simulink model "paper_model"  (R2021a)
settings: Solver=VariableStepAuto  StartTime=0.0  StopTime=720  RelTol=1e-3
libraries: fuzblock x2, mpcadaslib x1
settings Model: Creator=uddin  LastModifiedBy=uddin

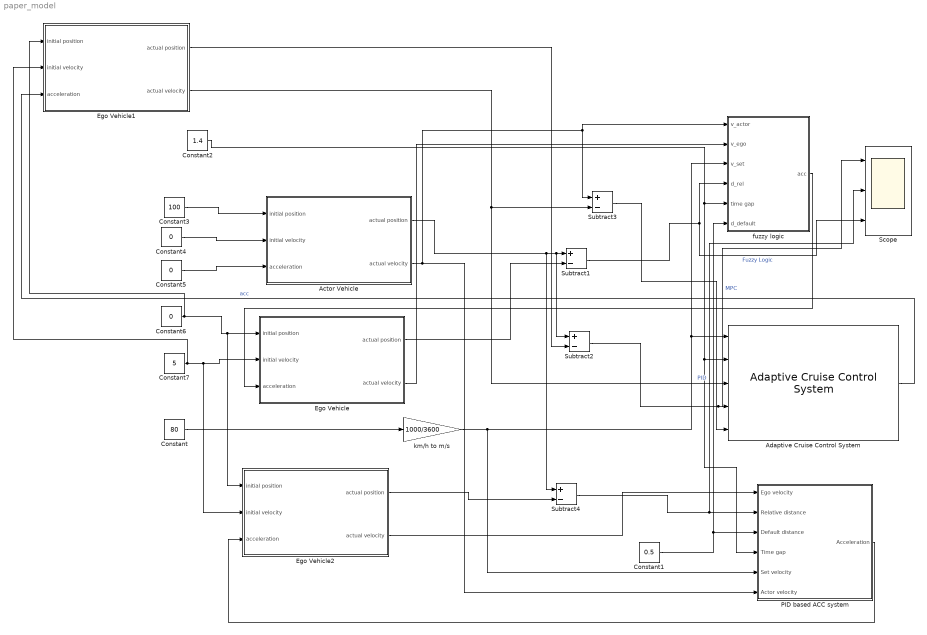
== system paper_model ==
  Actor Vehicle : Subsystem
  Adaptive Cruise Control System : mpcadaslib/Adaptive Cruise Control System  EgoModel=tf(1,[0.5,1,0])  InitialEgoVelocity=50*1000/3600  DefaultSpacing=0.5  MaxVelocity=120*1000/3600  MinAcceleration=-3  amin_ext=off  MaxAcceleration=2  amax_ext=off  Ts=.1  PredictionHorizon=100  ControllerBehavior=0.0  suboptimal=off  maxiter=10  datatypeopt=double  optmode=off  trackmode=off
  Constant : Constant  Value=80
  Constant1 : Constant  Value=0.5  SampleTime=-1
  Constant2 : Constant  Value=1.4  SampleTime=-1
  Constant3 : Constant  Value=100  SampleTime=-1
  Constant4 : Constant  Value=0  SampleTime=-1
  Constant5 : Constant  Value=0  SampleTime=-1
  Constant6 : Constant  Value=0  SampleTime=-1
  Constant7 : Constant  Value=5  SampleTime=-1
  Ego Vehicle : Subsystem
  Ego Vehicle1 : Subsystem
  Ego Vehicle2 : Subsystem
  PID based ACC system : Subsystem
  Scope : Scope  NumInputPorts=3
  Subtract{1..4} (4 alike) : Sum  Inputs=+-
  fuzzy logic : Subsystem
  km/h to m/s : Gain  Gain=1000/3600
  wires:
  Constant5/1 -> Actor Vehicle/3(acceleration)
  Constant3/1 -> Actor Vehicle/1(initial position)
  Constant6/1 -> Ego Vehicle1/1(initial position), Ego Vehicle2/1(initial position), Ego Vehicle/1(initial position)
  Constant7/1 -> Ego Vehicle1/2(initial velocity), Ego Vehicle2/2(initial velocity), Ego Vehicle/2(initial velocity)
  Constant4/1 -> Actor Vehicle/2(initial velocity)
  Actor Vehicle/1(actual position) -> Subtract4/1, Subtract2/1, Subtract1/1
  Actor Vehicle/2(actual velocity) -> PID based ACC system/6(Actor velocity), Subtract3/1, fuzzy logic/1(v_actor)
  Ego Vehicle/1(actual position) -> Subtract1/2
  fuzzy logic/1(acc) -> Ego Vehicle/3(acceleration)
  Subtract1/1 -> Scope/3, fuzzy logic/4(d_rel)  "Fuzzy Logic"
  Constant2/1 -> Adaptive Cruise Control System/2, PID based ACC system/4(Time gap), fuzzy logic/5(time gap)
  Constant/1 -> km/h to m/s/1
  km/h to m/s/1 -> PID based ACC system/5(Set velocity), Adaptive Cruise Control System/1, fuzzy logic/3(v_set)
  Ego Vehicle/2(actual velocity) -> fuzzy logic/2(v_ego)
  Ego Vehicle1/1(actual position) -> Subtract2/2
  Subtract2/1 -> Scope/1, Adaptive Cruise Control System/4  "MPC"
  Ego Vehicle1/2(actual velocity) -> Subtract3/2, Adaptive Cruise Control System/3
  Subtract3/1 -> Adaptive Cruise Control System/5
  Adaptive Cruise Control System/1 -> Ego Vehicle1/3(acceleration)  "acc"
  Ego Vehicle2/1(actual position) -> Subtract4/2
  Subtract4/1 -> PID based ACC system/2(Relative distance), Scope/2  "PID"
  PID based ACC system/1(Acceleration) -> Ego Vehicle2/3(acceleration)
  Ego Vehicle2/2(actual velocity) -> PID based ACC system/1(Ego velocity)
  Constant1/1 -> fuzzy logic/6(d_default), PID based ACC system/3(Default distance)

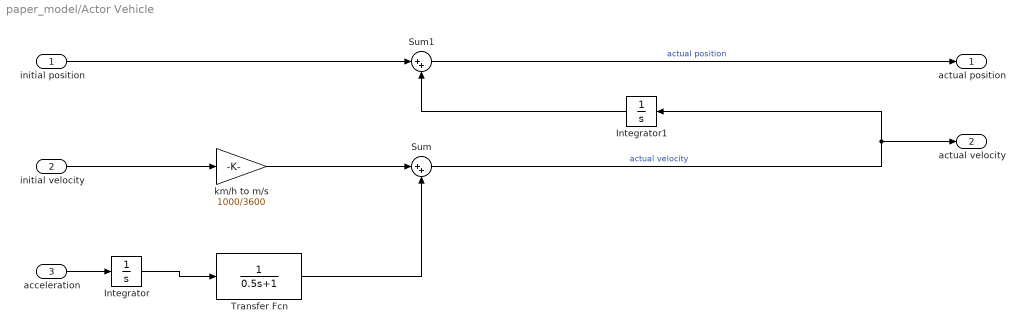
== system paper_model/Actor Vehicle ==
  initial position : Inport
  initial velocity : Inport  Port=2
  acceleration : Inport  Port=3
  Integrator : Integrator
  Integrator1 : Integrator
  Sum : Sum  Inputs=|++
  Sum1 : Sum  Inputs=|++
  Transfer Fcn : TransferFcn  Denominator=[0.5 1]
  km/h to m/s : Gain  Gain=1000/3600
  actual position : Outport
  actual velocity : Outport  Port=2
  wires:
  km/h to m/s/1 -> Sum/1
  initial velocity/1 -> km/h to m/s/1
  Transfer Fcn/1 -> Sum/2
  Integrator/1 -> Transfer Fcn/1
  Integrator1/1 -> Sum1/2
  initial position/1 -> Sum1/1
  acceleration/1 -> Integrator/1
  Sum/1 -> Integrator1/1, actual velocity/1  "actual velocity"
  Sum1/1 -> actual position/1  "actual position"

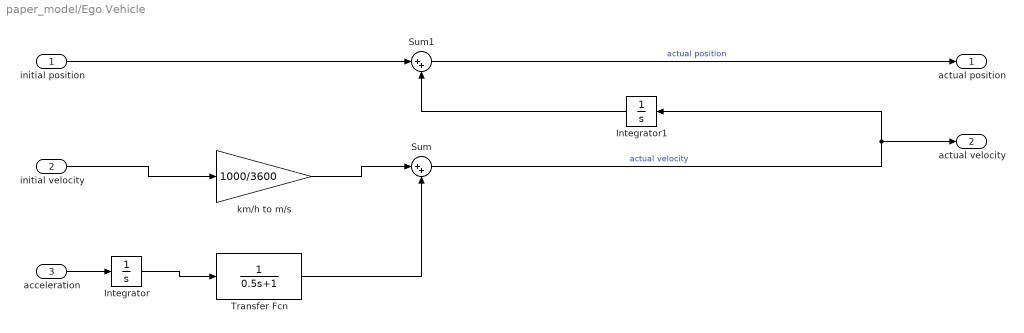
== system paper_model/Ego Vehicle ==
  initial position : Inport
  initial velocity : Inport  Port=2
  acceleration : Inport  Port=3
  Integrator : Integrator
  Integrator1 : Integrator
  Sum : Sum  Inputs=|++
  Sum1 : Sum  Inputs=|++
  Transfer Fcn : TransferFcn  Denominator=[0.5 1]
  km/h to m/s : Gain  Gain=1000/3600
  actual position : Outport
  actual velocity : Outport  Port=2
  wires:
  Sum1/1 -> actual position/1  "actual position"
  Sum/1 -> actual velocity/1, Integrator1/1  "actual velocity"
  acceleration/1 -> Integrator/1
  initial position/1 -> Sum1/1
  Integrator1/1 -> Sum1/2
  Integrator/1 -> Transfer Fcn/1
  Transfer Fcn/1 -> Sum/2
  initial velocity/1 -> km/h to m/s/1
  km/h to m/s/1 -> Sum/1

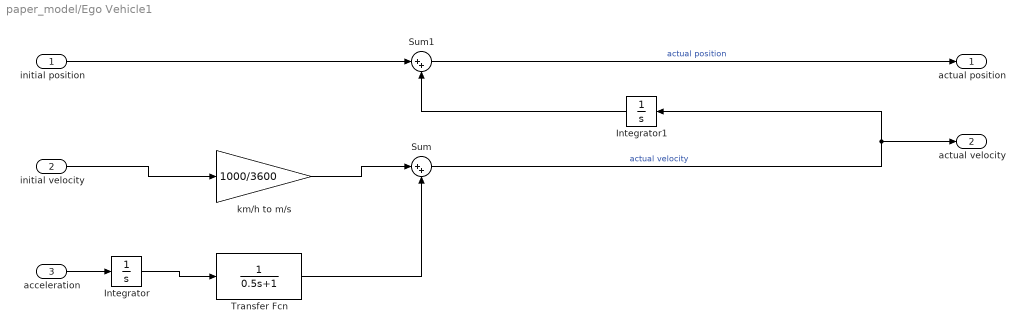
== system paper_model/Ego Vehicle1 ==
  initial position : Inport
  initial velocity : Inport  Port=2
  acceleration : Inport  Port=3
  Integrator : Integrator
  Integrator1 : Integrator
  Sum : Sum  Inputs=|++
  Sum1 : Sum  Inputs=|++
  Transfer Fcn : TransferFcn  Denominator=[0.5 1]
  km/h to m/s : Gain  Gain=1000/3600
  actual position : Outport
  actual velocity : Outport  Port=2
  wires:
  km/h to m/s/1 -> Sum/1
  initial velocity/1 -> km/h to m/s/1
  Transfer Fcn/1 -> Sum/2
  Integrator/1 -> Transfer Fcn/1
  Integrator1/1 -> Sum1/2
  initial position/1 -> Sum1/1
  acceleration/1 -> Integrator/1
  Sum/1 -> Integrator1/1, actual velocity/1  "actual velocity"
  Sum1/1 -> actual position/1  "actual position"

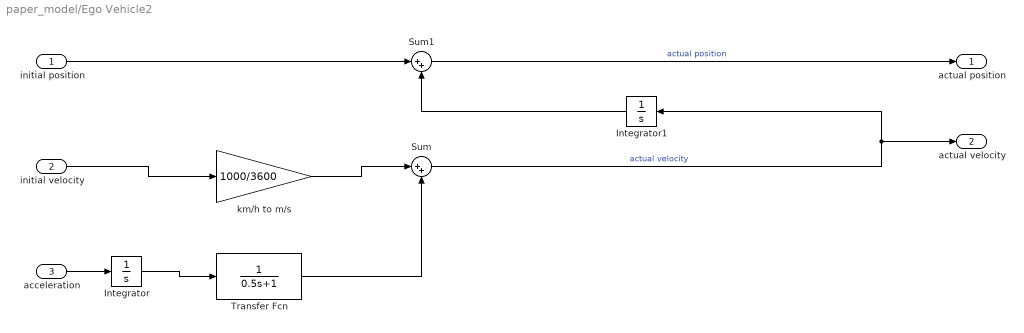
== system paper_model/Ego Vehicle2 ==
  initial position : Inport
  initial velocity : Inport  Port=2
  acceleration : Inport  Port=3
  Integrator : Integrator
  Integrator1 : Integrator
  Sum : Sum  Inputs=|++
  Sum1 : Sum  Inputs=|++
  Transfer Fcn : TransferFcn  Denominator=[0.5 1]
  km/h to m/s : Gain  Gain=1000/3600
  actual position : Outport
  actual velocity : Outport  Port=2
  wires:
  Sum1/1 -> actual position/1  "actual position"
  Sum/1 -> actual velocity/1, Integrator1/1  "actual velocity"
  acceleration/1 -> Integrator/1
  initial position/1 -> Sum1/1
  Integrator1/1 -> Sum1/2
  Integrator/1 -> Transfer Fcn/1
  Transfer Fcn/1 -> Sum/2
  initial velocity/1 -> km/h to m/s/1
  km/h to m/s/1 -> Sum/1

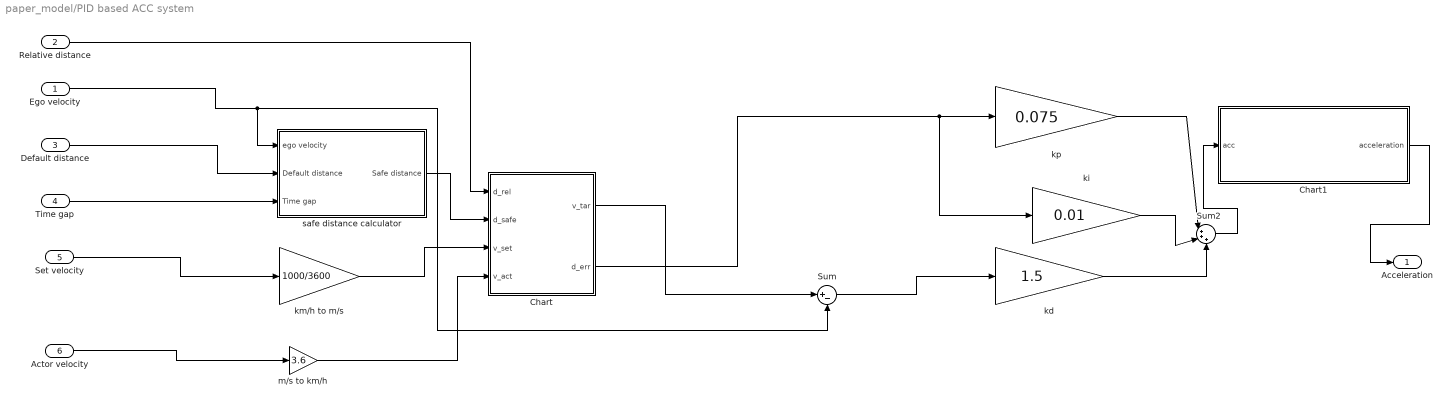
== system paper_model/PID based ACC system ==
  Ego velocity : Inport
  Relative distance : Inport  Port=2
  Default distance : Inport  Port=3
  Time gap : Inport  Port=4
  Set velocity : Inport  Port=5
  Actor velocity : Inport  Port=6
  Chart : Stateflow chart  TreatAsAtomicUnit=on
  Chart1 : Stateflow chart  TreatAsAtomicUnit=on
  Sum : Sum  Inputs=|+-
  Sum2 : Sum  Inputs=|+++
  kd : Gain  Gain=1.5
  ki : Gain  Gain=0.01
  km/h to m/s : Gain  Gain=1000/3600
  kp : Gain  Gain=0.075
  m/s to km/h : Gain  Gain=3.6
  safe distance calculator : Subsystem
  Acceleration : Outport
  wires:
  Default distance/1 -> safe distance calculator/2(Default distance)
  Set velocity/1 -> km/h to m/s/1
  Time gap/1 -> safe distance calculator/3(Time gap)
  Ego velocity/1 -> safe distance calculator/1(ego velocity), Sum/2
  kd/1 -> Sum2/3
  ki/1 -> Sum2/2
  kp/1 -> Sum2/1
  Relative distance/1 -> Chart/1(d_rel)
  safe distance calculator/1(Safe distance) -> Chart/2(d_safe)
  km/h to m/s/1 -> Chart/3(v_set)
  Sum2/1 -> Chart1/1(acc)
  Chart1/1(acceleration) -> Acceleration/1
  Sum/1 -> kd/1
  Chart/1(v_tar) -> Sum/1
  Chart/2(d_err) -> ki/1, kp/1
  Actor velocity/1 -> m/s to km/h/1
  m/s to km/h/1 -> Chart/4(v_act)

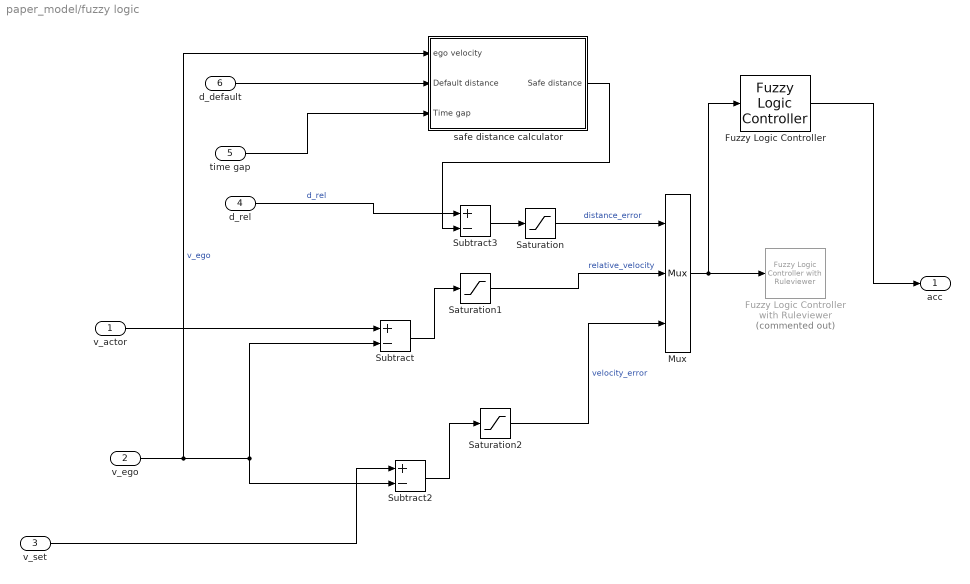
== system paper_model/fuzzy logic ==
  v_actor : Inport
  v_ego : Inport  Port=2
  v_set : Inport  Port=3
  d_rel : Inport  Port=4
  time gap : Inport  Port=5
  d_default : Inport  Port=6
  Fuzzy Logic Controller : fuzblock/Fuzzy Logic  Controller  FIS=self_created  OutputSampleNumber=181  DataType=double  FuzzifiedInputs=off  RuleFiringStrengths=off  RuleOutputs=off  AggregatedOutputs=off  SimulateUsing=Interpreted execution  OutOfRangeInputValueMessage=warning  NoRuleFiredMessage=warning  EmptyOutputFuzzySetMessage=warning
  Fuzzy Logic Controller with Ruleviewer : fuzblock/Fuzzy Logic  Controller  with Ruleviewer  Commented=on  fismatrix=self_created  Ts=2
  Mux : Mux  Inputs=3
  Saturation : Saturate  UpperLimit=1  LowerLimit=-1  LinearizeAsGain=off
  Saturation1 : Saturate  UpperLimit=1  LowerLimit=-1  LinearizeAsGain=off
  Saturation2 : Saturate  UpperLimit=1  LowerLimit=-1  LinearizeAsGain=off
  Subtract : Sum  Inputs=+-
  Subtract2 : Sum  Inputs=+-
  Subtract3 : Sum  Inputs=+-
  safe distance calculator : Subsystem
  acc : Outport
  wires:
  time gap/1 -> safe distance calculator/3(Time gap)
  Saturation1/1 -> Mux/2  "relative_velocity"
  Saturation2/1 -> Mux/3  "velocity_error"
  safe distance calculator/1(Safe distance) -> Subtract3/2
  Subtract3/1 -> Saturation/1
  v_ego/1 -> safe distance calculator/1(ego velocity), Subtract2/2, Subtract/2  "v_ego"
  Saturation/1 -> Mux/1  "distance_error"
  Mux/1 -> Fuzzy Logic Controller/1, Fuzzy Logic Controller with Ruleviewer/1
  Subtract/1 -> Saturation1/1
  Subtract2/1 -> Saturation2/1
  d_default/1 -> safe distance calculator/2(Default distance)
  d_rel/1 -> Subtract3/1  "d_rel"
  v_set/1 -> Subtract2/1
  v_actor/1 -> Subtract/1
  Fuzzy Logic Controller/1 -> acc/1

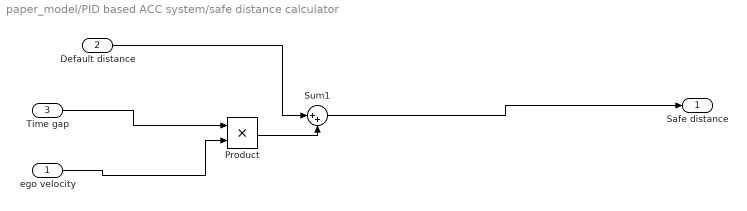
== system paper_model/PID based ACC system/safe distance calculator ==
  ego velocity : Inport
  Default distance : Inport  Port=2
  Time gap : Inport  Port=3
  Product : Product
  Sum1 : Sum  Inputs=|++
  Safe distance : Outport
  wires:
  Product/1 -> Sum1/2
  Sum1/1 -> Safe distance/1
  Time gap/1 -> Product/1
  Default distance/1 -> Sum1/1
  ego velocity/1 -> Product/2

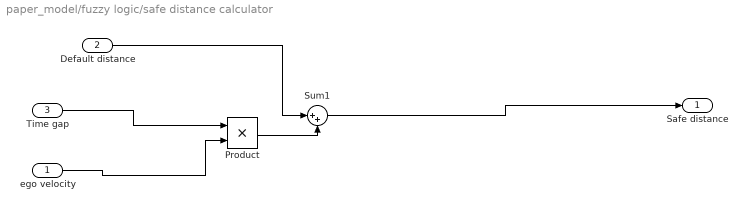
== system paper_model/fuzzy logic/safe distance calculator ==
  ego velocity : Inport
  Default distance : Inport  Port=2
  Time gap : Inport  Port=3
  Product : Product
  Sum1 : Sum  Inputs=|++
  Safe distance : Outport
  wires:
  Product/1 -> Sum1/2
  Sum1/1 -> Safe distance/1
  Time gap/1 -> Product/1
  Default distance/1 -> Sum1/1
  ego velocity/1 -> Product/2

== stateflow chart paper_model/PID based ACC system/Chart1 ==
  (default) -> (junction 11)
  (junction 11) -> (junction 12) [order 1] : [acc>=3]
  (junction 11) -> (junction 13) [order 2]
  (junction 12) -> (junction 17) : {acceleration=3;}
  (junction 13) -> (junction 14) [order 1] : [acc<=-2]
  (junction 13) -> (junction 15) [order 2] : {acceleration=acc;}
  (junction 14) -> (junction 16) : {acceleration=-2;}
  (junction 16) -> (junction 15)
  (junction 17) -> (junction 16)
  (junction 15) -> (junction 18)
  data: acc input; acceleration output

== stateflow chart paper_model/PID based ACC system/Chart ==
  (default) -> (junction 7)
  (junction 7) -> (junction 8) [order 1] : [d_rel>d_safe]
  (junction 7) -> (junction 9) [order 2] : {v_tar=v_act;d_err=d_rel-d_safe;}
  (junction 8) -> (junction 10) : {v_tar=v_set;}
  (junction 10) -> (junction 9)
  (junction 9) -> (junction 11)
  data: d_rel input; d_safe input; v_set input; v_act input; v_tar output; d_err output
